simulink model "physical_architecture"  (R2024b)
settings: Solver=VariableStepAuto  StartTime=0.0  StopTime=10.0  RelTol=1e-3
settings Model: Creator=upattacini  LastModifiedBy=mfussi
settings DataIOCC: SaveOutput=off  SignalLogging=off  DSMLogging=off  SaveTime=off
settings RTWCC: GPUComputeCapability=3.5

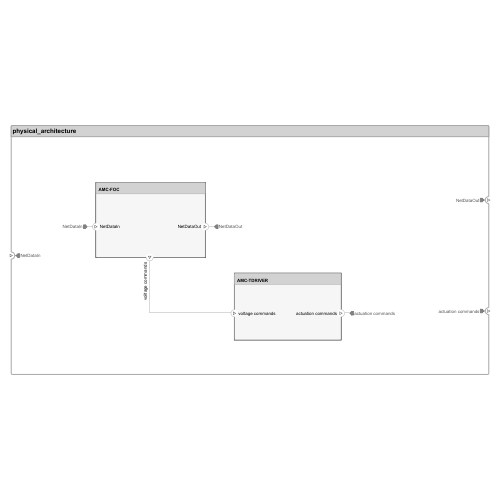
[thumbnail: Simulink's stored preview of the top-level diagram]
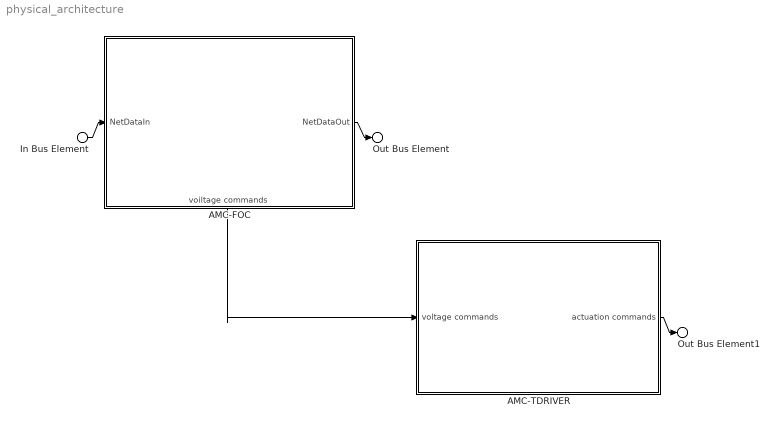
== system physical_architecture ==
  In Bus Element : Inport  PortName=NetDataIn
  AMC-FOC : Subsystem
      settings: PortSchema="{\"entries\":[{\"content\":{\"headerSize\":26,\"margin\":15,\"minimumSpacing\":25,\"sides\":[{\"content\":{\"connectorIds\":[\"In1\"]},\"type\":\"ConnectorPlacement.EquallySpacedRectSide\",\"uuid\":\"e347ee40-d54e-44fd-bc32-f8b024d9ce0e\"},{\"content\":{\"connectorIds\":[\"Out2\"],\"side\":\"RIGHT\"},\"type\":\"ConnectorPlacement.EquallySpacedRectSide\",\"uuid\":\"0804b9f8-7204-402a-a199-b5abf958a170\"},{\"content\":{\"side\":\"TOP\"},\"type\":\"ConnectorPlacement.EquallySpacedRectSide\",\"uuid\":\"09180045-bcf9-4b06-aaa4-a03943964dca\"},{\"content\":{\"connectorIds\":[\"Out1\"],\"side\":\"BOTTOM\"},\"type\":\"ConnectorPlacement.EquallySpacedRectSide\",\"uuid\":\"87c25ac9-9ca3-4ab9-a33c-eecd7d67217e\"}]},\"type\":\"ConnectorPlacement.EquallySpacedConnector\",\"uuid\":\"bea07901-0638-4912-923c-a7a96e6d9f8d\"}],\"packageUris\":[\"http://schema.mathworks.com/mf0/Connector/R2020b\"],\"version\":\"1.0\"}"
  AMC-TDRIVER : Subsystem
      settings: PortSchema="{\"entries\":[{\"content\":{\"headerSize\":26,\"margin\":15,\"minimumSpacing\":25,\"sides\":[{\"content\":{\"connectorIds\":[\"In1\"]},\"type\":\"ConnectorPlacement.EquallySpacedRectSide\",\"uuid\":\"e347ee40-d54e-44fd-bc32-f8b024d9ce0e\"},{\"content\":{\"connectorIds\":[\"Out1\"],\"side\":\"RIGHT\"},\"type\":\"ConnectorPlacement.EquallySpacedRectSide\",\"uuid\":\"0804b9f8-7204-402a-a199-b5abf958a170\"},{\"content\":{\"side\":\"TOP\"},\"type\":\"ConnectorPlacement.EquallySpacedRectSide\",\"uuid\":\"09180045-bcf9-4b06-aaa4-a03943964dca\"}]},\"type\":\"ConnectorPlacement.EquallySpacedConnector\",\"uuid\":\"bea07901-0638-4912-923c-a7a96e6d9f8d\"}],\"packageUris\":[\"http://schema.mathworks.com/mf0/Connector/R2020b\"],\"version\":\"1.0\"}"
  Out Bus Element : Outport  PortName=NetDataOut
  Out Bus Element1 : Outport  Port=2  PortName=actuation commands
  wires:
  In Bus Element/1 -> AMC-FOC/1(NetDataIn)
  AMC-FOC/2(NetDataOut) -> Out Bus Element/1
  AMC-FOC/1(voiltage commands) -> AMC-TDRIVER/1(voltage commands)
  AMC-TDRIVER/1(actuation commands) -> Out Bus Element1/1

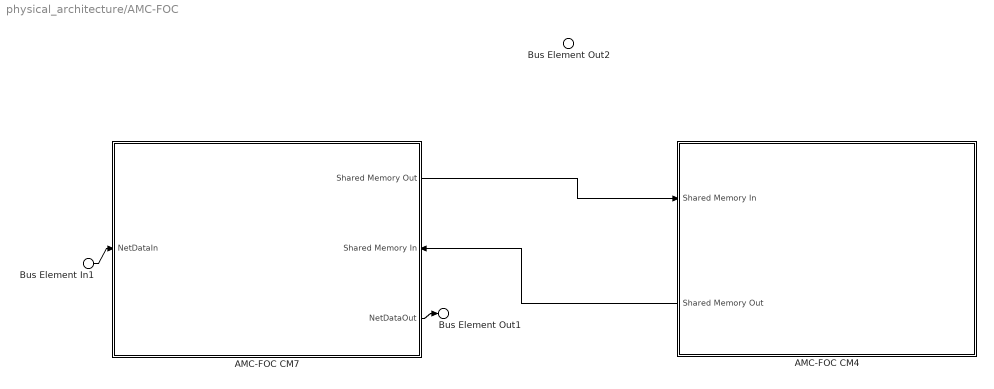
== system physical_architecture/AMC-FOC ==
  Bus Element In1 : Inport  PortName=NetDataIn
  AMC-FOC CM4 : Subsystem
      settings: PortSchema="{\"entries\":[{\"content\":{\"headerSize\":26,\"margin\":15,\"minimumSpacing\":25,\"sides\":[{\"content\":{\"connectorIds\":[\"In1\",\"Out1\"]},\"type\":\"ConnectorPlacement.EquallySpacedRectSide\",\"uuid\":\"e347ee40-d54e-44fd-bc32-f8b024d9ce0e\"},{\"content\":{\"side\":\"RIGHT\"},\"type\":\"ConnectorPlacement.EquallySpacedRectSide\",\"uuid\":\"0804b9f8-7204-402a-a199-b5abf958a170\"},{\"content\":{\"side\":\"TOP\"},\"type\":\"ConnectorPlacement.EquallySpacedRectSide\",\"uuid\":\"09180045-bcf9-4b06-aaa4-a03943964dca\"}]},\"type\":\"ConnectorPlacement.EquallySpacedConnector\",\"uuid\":\"bea07901-0638-4912-923c-a7a96e6d9f8d\"}],\"packageUris\":[\"http://schema.mathworks.com/mf0/Connector/R2020b\"],\"version\":\"1.0\"}"
  AMC-FOC CM7 : Subsystem
      settings: PortSchema="{\"entries\":[{\"content\":{\"headerSize\":26,\"margin\":15,\"minimumSpacing\":25,\"sides\":[{\"content\":{\"connectorIds\":[\"In2\"]},\"type\":\"ConnectorPlacement.EquallySpacedRectSide\",\"uuid\":\"e347ee40-d54e-44fd-bc32-f8b024d9ce0e\"},{\"content\":{\"connectorIds\":[\"Out1\",\"In1\",\"Out2\"],\"side\":\"RIGHT\"},\"type\":\"ConnectorPlacement.EquallySpacedRectSide\",\"uuid\":\"0804b9f8-7204-402a-a199-b5abf958a170\"},{\"content\":{\"side\":\"TOP\"},\"type\":\"ConnectorPlacement.EquallySpacedRectSide\",\"uuid\":\"09180045-bcf9-4b06-aaa4-a03943964dca\"}]},\"type\":\"ConnectorPlacement.EquallySpacedConnector\",\"uuid\":\"bea07901-0638-4912-923c-a7a96e6d9f8d\"}],\"packageUris\":[\"http://schema.mathworks.com/mf0/Connector/R2020b\"],\"version\":\"1.0\"}"
  Bus Element Out2 : Outport  PortName=voiltage commands
  Bus Element Out1 : Outport  Port=2  PortName=NetDataOut
  wires:
  Bus Element In1/1 -> AMC-FOC CM7/2(NetDataIn)
  AMC-FOC CM7/2(NetDataOut) -> Bus Element Out1/1
  AMC-FOC CM7/1(Shared Memory Out) -> AMC-FOC CM4/1(Shared Memory In)
  AMC-FOC CM4/1(Shared Memory Out) -> AMC-FOC CM7/1(Shared Memory In)

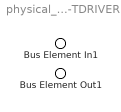
== system physical_architecture/AMC-TDRIVER ==
  Bus Element In1 : Inport  PortName=voltage commands
  Bus Element Out1 : Outport  PortName=actuation commands

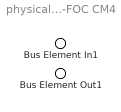
== system physical_architecture/AMC-FOC/AMC-FOC CM4 ==
  Bus Element In1 : Inport  PortName=Shared Memory In
  Bus Element Out1 : Outport  PortName=Shared Memory Out

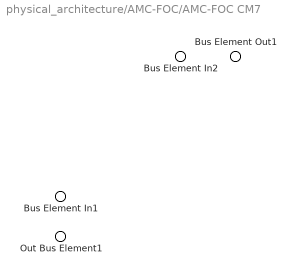
== system physical_architecture/AMC-FOC/AMC-FOC CM7 ==
  Bus Element In2 : Inport  PortName=Shared Memory In
  Bus Element In1 : Inport  Port=2  PortName=NetDataIn
  Bus Element Out1 : Outport  PortName=Shared Memory Out
  Out Bus Element1 : Outport  Port=2  PortName=NetDataOut
